simulink model "test_detectors"  (R2014a)
settings: Solver=FixedStepDiscrete  StartTime=0.0  StopTime=inf  FixedStep=SampleTime  RelTol=1e-3
settings Model: Creator=georg  LastModifiedBy=georg

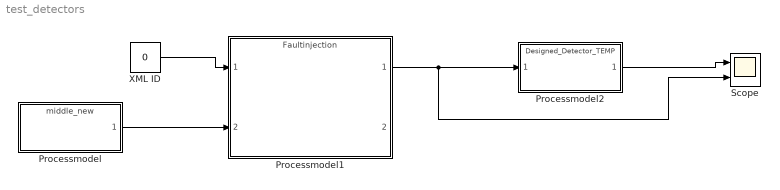
== system test_detectors ==
  Processmodel : ModelReference  ModelNameDialog=middle_new.slx  SimulationMode=Normal  ModelReferenceVersion=1.19  CopyOfModelName=middle_new.slx  DefaultDataLogging=on
  Processmodel1 : ModelReference  ModelNameDialog=Faultinjection.slx  SimulationMode=Normal  ModelReferenceVersion=1.10  CopyOfModelName=Faultinjection.slx  DefaultDataLogging=on
  Processmodel2 : ModelReference  ModelNameDialog=Designed_Detector_TEMP.slx  SimulationMode=Normal  ModelReferenceVersion=1.24  CopyOfModelName=Designed_Detector_TEMP.slx  DefaultDataLogging=on
  Scope : Scope  NumInputPorts=2
      settings: YMin=0~0  YMax=1~3.75
  XML ID : Constant  Value=0  OutDataTypeStr=single
  wires:
  Processmodel/1 -> Processmodel1/2
  XML ID/1 -> Processmodel1/1
  Processmodel1/1 -> Scope/2, Processmodel2/1
  Processmodel2/1 -> Scope/1
